simulink library "myLibrary"  (R2023a)
settings: Solver=VariableStepAuto  StartTime=0.0  StopTime=10.0  RelTol=1e-3
undefined symbols (not defined in the file): Cac_n1, ctrl1, Da, Discrete, dtha, ee_sli_rtmsupport, FA, gcbh, Ha, Ini, init_line, init_load, init_SG, init_TH, init_trafo, init_VSC, initMachineBlocks, Ka, Lf, Llkd_pu, Llkq1_pu, NET, P, plots_step, q0, Rac_n1, Radd, Rkd_pu, Rkq1_pu, Rload_add, sim_config, spsSteamTurbineModel, T_global, T_load, T_NET, T_SG, T_TH, T_trafo, T_VSC, Ts, tstep, V1
libraries: spsSeriesRLCBranchLib x57, spsParallelRLCBranchLib x39, eeGeneralControl x38, spsCurrentMeasurementLib x20, spsFirstOrderFilterLib x16, spsVoltageMeasurementLib x14, spsControlledVoltageSourceLib x12, $bdroot x9, dspsigops x6, spsThreePhaseVIMeasurementLib x5, spsPLL3phLib x4, spsThreePhaseBreakerLib x3
(part 1 of 7)
settings Model: Creator=CITCEA  LastModifiedBy=Francesca
settings DebuggingCC: UnconnectedInputMsg=warning  UnconnectedOutputMsg=warning  UnconnectedLineMsg=warning
settings ModelReferenceCC: EnableRefExpFcnMdlSchedulingChecks=on
settings RTWCC: DLArmComputeVersion=19.05

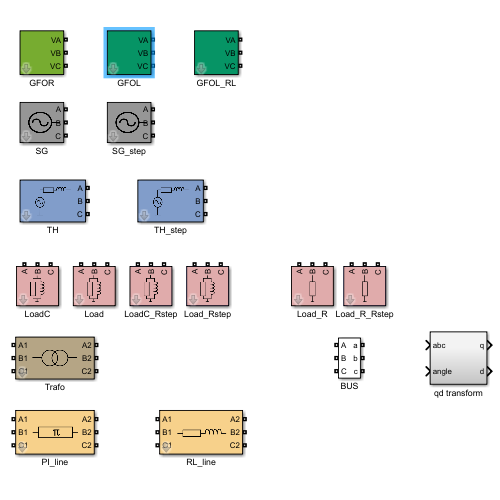
[thumbnail: Simulink's stored preview of the top-level diagram]
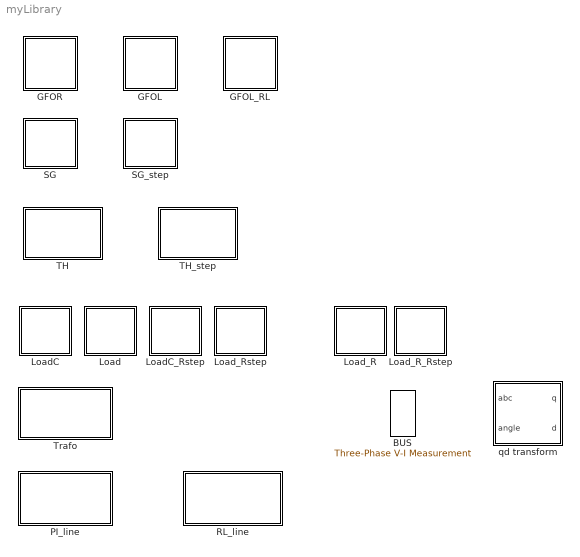
== system myLibrary ==
  BUS : spsThreePhaseVIMeasurementLib/Three-Phase V-I Measurement  VoltageMeasurement=phase-to-phase  SetLabelV=on  LabelV=V  Vpu=off  VpuLL=off  CurrentMeasurement=yes  SetLabelI=on  LabelI=I  Ipu=off  Pbase=100e6  Vbase=500e3  OutputType=Complex  PhasorSimulation=off  PSBequivalent=0
  GFOL : Subsystem  mask{T_VSC_global=T_VSC, initVSC_global=init_VSC, num=1}
      mask prompts: T_VSC_global "T_VSC"; initVSC_global "init_VSC"
      mask init:
      | T_VSC = T_VSC_global(num,:);
      | initVSC = initVSC_global{num};
      | 
      | set_param([gcb '/Control/Goto_w'],'GotoTag',['w_GFOL' num2str(num)])
      | set_param([gcb '/Control/From_w'],'GotoTag',['w_GFOL' num2str(num)])
  GFOL_RL : Subsystem  mask{T_VSC_global=T_VSC, initVSC_global=init_VSC, num=1}
      mask prompts: T_VSC_global "T_VSC"; initVSC_global "init_VSC"
      mask init:
      | T_VSC = T_VSC_global(num,:);
      | initVSC = initVSC_global{num};
      | 
      | set_param([gcb '/Control/Goto_w'],'GotoTag',['w_GFOL' num2str(num)])
      | set_param([gcb '/Control/From_w'],'GotoTag',['w_GFOL' num2str(num)])
  GFOR : Subsystem  mask{T_VSC_global=T_VSC, initVSC_global=init_VSC, num=1}
      mask prompts: T_VSC_global "T_VSC"; initVSC_global "init_VSC"
      mask init:
      | T_VSC = T_VSC_global(num,:);
      | initVSC = initVSC_global{num};
      | 
      | set_param([gcb '/Control/Goto_theta'],'GotoTag',['theta_GFOR' num2str(num)])
      | set_param([gcb '/Control/PLL/Goto_w'],'GotoTag',['w_GFOR' num2str(num)])
  Load : Subsystem  mask{T_load_global=T_load, initLoad_global=init_load, num=1}
      mask prompts: T_load_global "T_load"; initLoad_global "init_load"
      mask init:
      | T = T_load_global(num,:);
      | ini = initLoad_global{num};
      mask Display:
      | % Use specified image as mask icon
      | image('load.png')
  LoadC : Subsystem  mask{T_load_global=T_load, initLoad_global=init_load, num=1}
      mask prompts: T_load_global "T_load"; initLoad_global "init_load"
      mask init:
      | T = T_load_global(num,:);
      | ini = initLoad_global{num};
      mask Display:
      | % Use specified image as mask icon
      | image('load.png')
  LoadC_Rstep : Subsystem  mask{T_load_global=T_load, initLoad_global=init_load, num=1, tstep=tstep, Radd=Radd}
      mask prompts: T_load_global "T_load"; initLoad_global "init_load"
      mask init:
      | T = T_load_global(num,:);
      | ini = initLoad_global{num};
      mask Display:
      | % Use specified image as mask icon
      | image('load.png')
  Load_R : Subsystem  mask{T_load_global=T_load, num=1}
      mask prompts: T_load_global "T_load"
      mask init:
      | T = T_load_global(num,:);
      mask Display:
      | % Use specified image as mask icon
      | image('load_R.png')
  Load_R_Rstep : Subsystem  mask{T_load_global=T_load, num=1, tstep=tstep, Radd=Radd}
      mask prompts: T_load_global "T_load"
      mask init:
      | T = T_load_global(num,:);
      mask Display:
      | % Use specified image as mask icon
      | image('load_R.png')
  Load_Rstep : Subsystem  mask{T_load_global=T_load, initLoad_global=init_load, num=1, tstep=tstep, Radd=Radd}
      mask prompts: T_load_global "T_load"; initLoad_global "init_load"
      mask init:
      | T = T_load_global(num,:);
      | ini = initLoad_global{num};
      mask Display:
      | % Use specified image as mask icon
      | image('load.png')
  PI_line : Subsystem  mask{T_line_global=T_NET, initLine_global=init_line, num=1, set_C0=ones(1,6), set_iL0=0}
      mask prompts: T_line_global "T_line"; initLine_global "init_line"; set_C0 "init_cap"; set_iL0 "init_ind"
      mask init:
      | T = T_line_global(num,:);
      | ini = initLine_global{num};
      | set_C00 = set_C0(1,1);
      | set_C01 = set_C0(1,2);
      | set_C02 = set_C0(1,3);
      | set_C03 = set_C0(1,4);
      | set_C04 = set_C0(1,5);
      | set_C05 = set_C0(1,6);
      | set_param([gcb '/Series RLC Branch'],'Setx0',set_C00)
      | set_param([gcb '/Series RLC Branch1'],'Setx0',set_C01)
      | set_param([gcb '/Series RLC Branch2'],'Setx0',set_C02)
      | set_param([gcb '/Series RLC Branch3'],'Setx0',set_C03)
      | set_param([gcb '/Series RLC Branch4'],'Setx0',set_C04)
      | set_param([gcb '/Series RLC Branch5'],'Setx0',set_C05)
      | set_param([gcb '/Series RLC Branch6'],'SetiL0',set_iL0)
      mask Display:
      | % Use specified image as mask icon
      | image('PI.png')
  RL_line : Subsystem  mask{T_line_global=T_NET, initLine_global=init_line, num=1}
      mask prompts: T_line_global "T_line"; initLine_global "init_line"
      mask init:
      | T = T_line_global(num,:);
      | ini = initLine_global{num};
      mask Display:
      | % Use specified image as mask icon
      | image('RL.png')
  SG : Subsystem  mask{num=1, init_SG_global=init_SG, initMachineBlocks=initMachineBlocks, T_SG_global=T_SG}
      mask prompts: init_SG_global "init_SG"; initMachineBlocks "initMachine"; T_SG_global "T_SG"
      mask init:
      | initSG = init_SG_global{num};
      | T_SG = T_SG_global(num,:);
      | SGnum = num;
      | 
      | T_SG.exc = T_SG.exc{:};
      | T_SG.mech = T_SG.mech{:};
      | T_SG.PSS = T_SG.PSS{:};
      | 
      | 
      | switch T_SG.pss{:}
      |     case '2A'
      |         hasPSS = 1;
      |         set_param([gcb '/Exciter/PSS 2A'],'commented', 'off')
      |     case 'no'
      |         hasPSS = 0;
      |         set_param([gcb '/Exciter/PSS 2A'],'commented', 'on')
      | end
      | 
      | switch T_SG.govturb{:}
      |     case 'IEEEG1'
      |         selectGovturb= 1;
      |         set_param([gcb '/Governor-Turbine/IEEEG1'],'commented', 'off')
      |         set_param([gcb '/Governor-Turbine/Steam Turbine and Governor'],'commented', 'on')
      |     case 'TANDEM-SINGLE'
      |         selectGovturb= 2;
      |         T_SG.genType = 0;
      |         set_param([gcb '/Governor-Turbine/IEEEG1'],'commented', 'on')
      |         set_param([gcb '/Governor-Turbine/Steam Turbine and Governor'],'commented', 'off')
      |     case 'TANDEM-MULTI'
      |         selectGovturb= 2;
      |         T_SG.genType = 1;
      |         set_param([gcb '/Governor-Turbine/IEEEG1'],'commented', 'on')
      |         set_param([gcb '/Governor-Turbine/Steam Turbine and Governor'],'commented', 'off')
      |     case 'no'
      |         selectGovturb= 3;
      |         set_param([gcb '/Governor-Turbine/IEEEG1'],'commented', 'on')
      |         set_param([gcb '/Governor-Turbine/Steam Turbine and Governor'],'commented', 'on')
      | end
      | 
      | switch T_SG.exciter{:} 
      |     case 'AC4A'
      |         selectExciter = 1;
      |         set_param([gcb '/Exciter/Exciter AC4A'],'commented', 'off')
      |         set_param([gcb '/Exciter/Exciter ST4B'],'commented', 'on')
      |         set_param([gcb '/Exciter/Exciter ST1'],'commented', 'on')
      |     case 'ST4B'
      |         selectExciter = 2;
      |         set_param([gcb '/Exciter/Exciter AC4A'],'commented', 'on')
      |         set_param([gcb '/Exciter/Exciter ST4B'],'commented', 'off')
      |         set_param([gcb '/Exciter/Exciter ST1'],'commented', 'on')
      |     case 'ST1'
      |         selectExciter = 3;
      |         set_param([gcb '/Exciter/Exciter AC4A'],'commented', 'on')
      |         set_param([gcb '/Exciter/Exciter ST4B'],'commented', 'on')
      |         set_param([gcb '/Exciter/Exciter ST1'],'commented', 'off')
      |     case 'no'
      |         selectExciter = 4;
      |         set_param([gcb '/Exciter/Exciter AC4A'],'commented', 'on')
      |         set_param([gcb '/Exciter/Exciter ST4B'],'commented', 'on')
      |         set_param([gcb '/Exciter/Exciter ST1'],'commented', 'on')
      | end
      | 
      | set_param([gcb '/Goto_theta'],'GotoTag',['theta_SG' num2str(SGnum)])
      | set_param([gcb '/Goto_w'],'GotoTag',['w_SG' num2str(SGnum)])
      mask Display:
      | % Use specified image as mask icon
      | image('SG.png')
  SG_step : Subsystem  mask{num=1, init_SG_global=init_SG, initMachineBlocks=initMachineBlocks, T_SG_global=T_SG, step_var=Pref, tstep=sim_config.tstep}
      mask prompts: init_SG_global "init_SG"; initMachineBlocks "initMachine"; T_SG_global "T_SG"
      mask init:
      | initSG = init_SG_global{num};
      | T_SG = T_SG_global(num,:);
      | SGnum = num;
      | 
      | T_SG.exc = T_SG.exc{:};
      | T_SG.mech = T_SG.mech{:};
      | T_SG.PSS = T_SG.PSS{:};
      | 
      | 
      | switch T_SG.pss{:}
      |     case '2A'
      |         hasPSS = 1;
      |         set_param([gcb '/Exciter/PSS 2A'],'commented', 'off')
      |     case 'no'
      |         hasPSS = 0;
      |         set_param([gcb '/Exciter/PSS 2A'],'commented', 'on')
      | end
      | 
      | switch T_SG.govturb{:}
      |     case 'IEEEG1'
      |         selectGovturb= 1;
      |         set_param([gcb '/Governor-Turbine/IEEEG1'],'commented', 'off')
      |         set_param([gcb '/Governor-Turbine/Steam Turbine and Governor'],'commented', 'on')
      |     case 'TANDEM-SINGLE'
      |         selectGovturb= 2;
      |         T_SG.genType = 0;
      |         set_param([gcb '/Governor-Turbine/IEEEG1'],'commented', 'on')
      |         set_param([gcb '/Governor-Turbine/Steam Turbine and Governor'],'commented', 'off')
      |     case 'TANDEM-MULTI'
      |         selectGovturb= 2;
      |         T_SG.genType = 1;
      |         set_param([gcb '/Governor-Turbine/IEEEG1'],'commented', 'on')
      |         set_param([gcb '/Governor-Turbine/Steam Turbine and Governor'],'commented', 'off')
      |     case 'no'
      |         selectGovturb= 3;
      |         set_param([gcb '/Governor-Turbine/IEEEG1'],'commented', 'on')
      |         set_param([gcb '/Governor-Turbine/Steam Turbine and Governor'],'commented', 'on')
      | end
      | 
      | switch T_SG.exciter{:} 
      |     case 'AC4A'
      |         selectExciter = 1;
      |         set_param([gcb '/Exciter/Exciter AC4A'],'commented', 'off')
      |         set_param([gcb '/Exciter/Exciter ST4B'],'commented', 'on')
      |         set_param([gcb '/Exciter/Exciter ST1'],'commented', 'on')
      |     case 'ST4B'
      |         selectExciter = 2;
      |         set_param([gcb '/Exciter/Exciter AC4A'],'commented', 'on')
      |         set_param([gcb '/Exciter/Exciter ST4B'],'commented', 'off')
      |         set_param([gcb '/Exciter/Exciter ST1'],'commented', 'on')
      |     case 'ST1'
      |         selectExciter = 3;
      |         set_param([gcb '/Exciter/Exciter AC4A'],'commented', 'on')
      |         set_param([gcb '/Exciter/Exciter ST4B'],'commented', 'on')
      |         set_param([gcb '/Exciter/Exciter ST1'],'commented', 'off')
      |     case 'no'
      |         selectExciter = 4;
      |         set_param([gcb '/Exciter/Exciter AC4A'],'commented', 'on')
      |         set_param([gcb '/Exciter/Exciter ST4B'],'commented', 'on')
      |         set_param([gcb '/Exciter/Exciter ST1'],'commented', 'on')
      | end
      | 
      | set_param([gcb '/Goto_theta'],'GotoTag',['theta_SG' num2str(SGnum)])
      | set_param([gcb '/Goto_w'],'GotoTag',['w_SG' num2str(SGnum)])
      | 
      | switch step_var
      |     case 'Pref'
      |         tstep_P = tstep;
      |         tstep_V = 1e3;
      |     case 'Vref'
      |         tstep_P = 1e3;
      |         tstep_V = tstep;
      | end
      mask TypeOptions step_var: Pref | Vref
      mask Display:
      | % Use specified image as mask icon
      | image('SG.png')
  TH : Subsystem  mask{T_TH_global=T_TH, initTH_global=init_TH, num=1}
      mask prompts: T_TH_global "T_TH"; initTH_global "init_TH"
      mask init:
      | T = T_TH_global(num,:);
      | ini = initTH_global{num};
      mask Display:
      | port_label('rconn', 1, 'A')
      | port_label('rconn', 2, 'B')
      | port_label('rconn', 3, 'C')
      | 
      | % Use specified image as mask icon
      | image('TH.png')
  TH_step : Subsystem  mask{T_TH_global=T_TH, initTH_global=init_TH, num=1, tstep=tstep, V1=V1}
      mask prompts: T_TH_global "T_TH"; initTH_global "init_TH"
      mask init:
      | T = T_TH_global(num,:);
      | ini = initTH_global{num};
      mask Display:
      | port_label('rconn', 1, 'A')
      | port_label('rconn', 2, 'B')
      | port_label('rconn', 3, 'C')
      | 
      | % Use specified image as mask icon
      | image('TH.png')
  Trafo : Subsystem  mask{T_trafo_global=T_trafo, initTrafo_global=init_trafo, num=3}
      mask prompts: T_trafo_global "T_trafo"; initTrafo_global "init_trafo"
      mask init:
      | T = T_trafo_global(num,:);
      | ini = initTrafo_global{num};
      mask Display:
      | % Use specified image as mask icon
      | image('trafo.png')
  qd transform : Subsystem

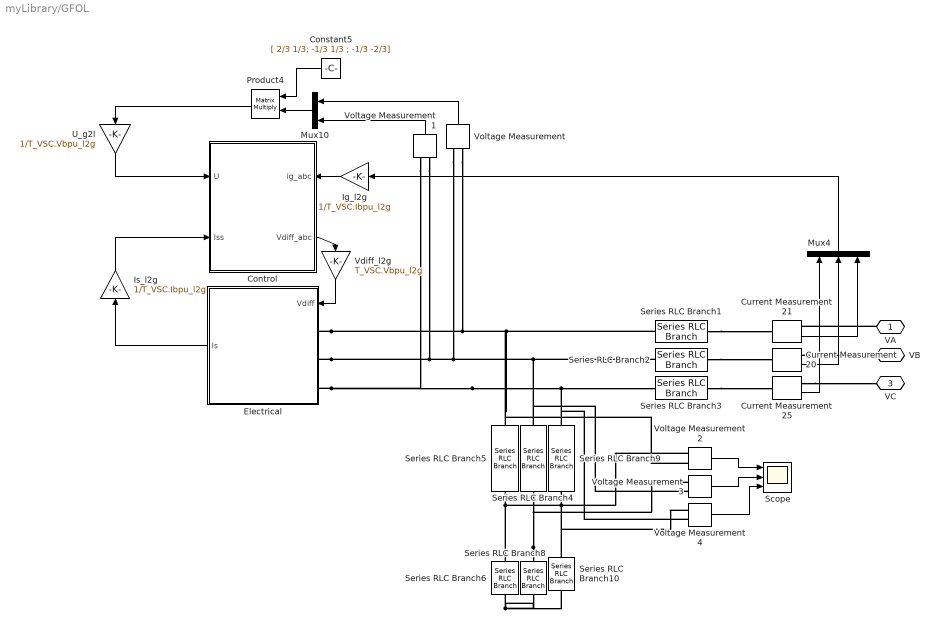
== system myLibrary/GFOL ==
  Constant5 : Constant  Value=[ 2/3 1/3; -1/3 1/3 ; -1/3 -2/3]
  Control : Subsystem
      settings: PortSchema="{\"entries\":[{\"content\":{\"sides\":[{\"content\":{},\"type\":\"ConnectorPlacement.EquallySpacedRectSide\",\"uuid\":\"681c0b5f-022d-4b6d-8fe2-73940743a76e\"},{\"content\":{\"side\":\"RIGHT\"},\"type\":\"ConnectorPlacement.EquallySpacedRectSide\",\"uuid\":\"e9b400c8-e13f-4caf-91a1-f348979675fd\"},{\"content\":{\"connectorIds\":[\"In1\",\"Out1\"],\"side\":\"TOP\"},\"type\":\"ConnectorPlacement.EquallySpacedRectSide\",\"uuid\":\"348007cb-ce67-4c45-ad7b-36ba89db6185\"},{\"content\":{\"connectorIds\":[\"In2\",\"In3\"],\"side\":\"BOTTOM\"},\"type\":\"ConnectorPlacement.EquallySpacedRectSide\",\"uuid\":\"fd6a847a-5d69-44cd-a0d1-495126761350\"}]},\"type\":\"ConnectorPlacement.EquallySpacedConnector\",\"uuid\":\"d16b8cae-5ced-4c76-a87e-983e154fb48f\"}],\"packageUris\":[\"http://schema.mathworks.com/mf0/Connector/R2020b\"],\"version\":\"1.0\"}"
  Current Measurement20 : spsCurrentMeasurementLib/Current Measurement  PhasorSimulation=off  OutputType=Complex  PSBequivalent=0
  Current Measurement21 : spsCurrentMeasurementLib/Current Measurement  PhasorSimulation=off  OutputType=Complex  PSBequivalent=0
  Current Measurement25 : spsCurrentMeasurementLib/Current Measurement  PhasorSimulation=off  OutputType=Complex  PSBequivalent=0
  Electrical : Subsystem
  Ig_l2g : Gain  Gain=1/T_VSC.Ibpu_l2g
  Is_l2g : Gain  Gain=1/T_VSC.Ibpu_l2g
  Mux10 : Mux  Inputs=2
  Mux4 : Mux  Inputs=3
  Product4 : Product  Multiplication=Matrix(*)
  Scope : Scope  NumInputPorts=3
  Series RLC Branch1 : spsSeriesRLCBranchLib/Series RLC Branch  LConnTagsString=__new0  RConnTagsString=__new0  BranchType=RL  Resistance=initVSC.Rtr  Inductance=initVSC.Ltr  SetiL0=off  InitialCurrent=initVSC.Iga  Capacitance=P.C  Setx0=on  InitialVoltage=P.C  Measurements=None
  Series RLC Branch10 : spsSeriesRLCBranchLib/Series RLC Branch  LConnTagsString=__new0  RConnTagsString=__new0  BranchType=R  Resistance=initVSC.Rac  Inductance=Lf  SetiL0=off  InitialCurrent=0  Capacitance=Cac_n1  Setx0=on  InitialVoltage=vcini_n1  Measurements=None
  Series RLC Branch2 : spsSeriesRLCBranchLib/Series RLC Branch  LConnTagsString=__new0  RConnTagsString=__new0  BranchType=RL  Resistance=initVSC.Rtr  Inductance=initVSC.Ltr  SetiL0=on  InitialCurrent=initVSC.Igb  Capacitance=P.C  Setx0=on  InitialVoltage=P.C  Measurements=None
  Series RLC Branch3 : spsSeriesRLCBranchLib/Series RLC Branch  LConnTagsString=__new0  RConnTagsString=__new0  BranchType=RL  Resistance=initVSC.Rtr  Inductance=initVSC.Ltr  SetiL0=on  InitialCurrent=initVSC.Igc  Capacitance=P.C  Setx0=on  InitialVoltage=P.C  Measurements=None
  Series RLC Branch4 : spsSeriesRLCBranchLib/Series RLC Branch  LConnTagsString=__new0  RConnTagsString=__new0  BranchType=C  Resistance=Rac_n1  Inductance=Lf  SetiL0=off  InitialCurrent=0  Capacitance=initVSC.Cac  Setx0=on  InitialVoltage=initVSC.Ucap_b  Measurements=None
  Series RLC Branch5 : spsSeriesRLCBranchLib/Series RLC Branch  LConnTagsString=__new0  RConnTagsString=__new0  BranchType=C  Resistance=Rac_n1  Inductance=Lf  SetiL0=off  InitialCurrent=0  Capacitance=initVSC.Cac  Setx0=on  InitialVoltage=initVSC.Ucap_a  Measurements=None
  Series RLC Branch6 : spsSeriesRLCBranchLib/Series RLC Branch  LConnTagsString=__new0  RConnTagsString=__new0  BranchType=R  Resistance=initVSC.Rac  Inductance=Lf  SetiL0=off  InitialCurrent=0  Capacitance=Cac_n1  Setx0=on  InitialVoltage=vcini_n1  Measurements=None
  Series RLC Branch8 : spsSeriesRLCBranchLib/Series RLC Branch  LConnTagsString=__new0  RConnTagsString=__new0  BranchType=R  Resistance=initVSC.Rac  Inductance=Lf  SetiL0=off  InitialCurrent=0  Capacitance=Cac_n1  Setx0=on  InitialVoltage=vcini_n1  Measurements=None
  Series RLC Branch9 : spsSeriesRLCBranchLib/Series RLC Branch  LConnTagsString=__new0  RConnTagsString=__new0  BranchType=C  Resistance=Rac_n1  Inductance=Lf  SetiL0=off  InitialCurrent=0  Capacitance=initVSC.Cac  Setx0=on  InitialVoltage=initVSC.Ucap_c  Measurements=None
  U_g2l : Gain  Gain=1/T_VSC.Vbpu_l2g
  Vdiff_l2g : Gain  Gain=T_VSC.Vbpu_l2g
  Voltage Measurement{,1..4} (5 alike) : spsVoltageMeasurementLib/Voltage Measurement  PhasorSimulation=off  OutputType=Complex  PSBequivalent=0
  VA : PMIOPort  Side=Right
  VB : PMIOPort  Port=2  Side=Right
  VC : PMIOPort  Port=3  Side=Right
  wires:
  Voltage Measurement4/1 -> Scope/3
  Voltage Measurement2/1 -> Scope/1
  Voltage Measurement3/1 -> Scope/2
  Ig_l2g/1 -> Control/1(ig_abc)
  Current Measurement25/1 -> Mux4/3
  Mux4/1 -> Ig_l2g/1
  Current Measurement21/1 -> Mux4/1
  Current Measurement20/1 -> Mux4/2
  U_g2l/1 -> Control/2(U)
  Is_l2g/1 -> Control/3(Iss)
  Vdiff_l2g/1 -> Electrical/1(Vdiff)
  Electrical/1(Is) -> Is_l2g/1
  Control/1(Vdiff_abc) -> Vdiff_l2g/1
  Product4/1 -> U_g2l/1
  Voltage Measurement/1 -> Mux10/1
  Mux10/1 -> Product4/2
  Constant5/1 -> Product4/1
  Voltage Measurement1/1 -> Mux10/2
  connections:
  Series RLC Branch6/RConn1 -- Series RLC Branch8/RConn1 -- Series RLC Branch10/RConn1
  Series RLC Branch9/RConn1 -- Series RLC Branch10/LConn1 -- Voltage Measurement4/LConn2
  Series RLC Branch8/LConn1 -- Series RLC Branch4/RConn1 -- Voltage Measurement3/LConn2
  Series RLC Branch5/RConn1 -- Series RLC Branch6/LConn1 -- Voltage Measurement2/LConn2
  Series RLC Branch3/RConn1 -- Current Measurement25/LConn1
  Series RLC Branch2/RConn1 -- Current Measurement20/LConn1
  Series RLC Branch1/RConn1 -- Current Measurement21/LConn1
  Current Measurement25/RConn1 -- VC/RConn1
  Electrical/LConn2 -- Voltage Measurement/LConn2 -- Series RLC Branch2/LConn1 -- Voltage Measurement3/LConn1 -- Series RLC Branch4/LConn1 -- Voltage Measurement1/LConn1
  VA/RConn1 -- Current Measurement21/RConn1
  Electrical/LConn3 -- Series RLC Branch3/LConn1 -- Voltage Measurement4/LConn1 -- Series RLC Branch9/LConn1 -- Voltage Measurement1/LConn2
  Electrical/LConn1 -- Voltage Measurement/LConn1 -- Voltage Measurement2/LConn1 -- Series RLC Branch5/LConn1 -- Series RLC Branch1/LConn1
  VB/RConn1 -- Current Measurement20/RConn1

== system myLibrary/GFOL_RL ==
  Constant5 : Constant  Value=[ 2/3 1/3; -1/3 1/3 ; -1/3 -2/3]
  Control : Subsystem
      settings: PortSchema="{\"entries\":[{\"content\":{\"sides\":[{\"content\":{\"connectorIds\":[]},\"type\":\"ConnectorPlacement.EquallySpacedRectSide\",\"uuid\":\"681c0b5f-022d-4b6d-8fe2-73940743a76e\"},{\"content\":{\"connectorIds\":[],\"side\":\"RIGHT\"},\"type\":\"ConnectorPlacement.EquallySpacedRectSide\",\"uuid\":\"e9b400c8-e13f-4caf-91a1-f348979675fd\"},{\"content\":{\"connectorIds\":[\"Out1\"],\"side\":\"TOP\"},\"type\":\"ConnectorPlacement.EquallySpacedRectSide\",\"uuid\":\"348007cb-ce67-4c45-ad7b-36ba89db6185\"},{\"content\":{\"connectorIds\":[\"In1\",\"In2\"],\"side\":\"BOTTOM\"},\"type\":\"ConnectorPlacement.EquallySpacedRectSide\",\"uuid\":\"fd6a847a-5d69-44cd-a0d1-495126761350\"}]},\"type\":\"ConnectorPlacement.EquallySpacedConnector\",\"uuid\":\"d16b8cae-5ced-4c76-a87e-983e154fb48f\"}],\"packageUris\":[\"http://schema.mathworks.com/mf0/Connector/R2020b\"],\"version\":\"1.0\"}"
  Electrical : Subsystem
  Is_l2g : Gain  Gain=1/T_VSC.Ibpu_l2g
  Mux10 : Mux  Inputs=2
  Product4 : Product  Multiplication=Matrix(*)
  Series RLC Branch1 : spsSeriesRLCBranchLib/Series RLC Branch  LConnTagsString=__new0  RConnTagsString=__new0  BranchType=RL  Resistance=initVSC.Rtr  Inductance=initVSC.Ltr  SetiL0=off  InitialCurrent=initVSC.Iga  Capacitance=P.C  Setx0=on  InitialVoltage=P.C  Measurements=None
  Series RLC Branch2 : spsSeriesRLCBranchLib/Series RLC Branch  LConnTagsString=__new0  RConnTagsString=__new0  BranchType=RL  Resistance=initVSC.Rtr  Inductance=initVSC.Ltr  SetiL0=on  InitialCurrent=initVSC.Igb  Capacitance=P.C  Setx0=on  InitialVoltage=P.C  Measurements=None
  Series RLC Branch3 : spsSeriesRLCBranchLib/Series RLC Branch  LConnTagsString=__new0  RConnTagsString=__new0  BranchType=RL  Resistance=initVSC.Rtr  Inductance=initVSC.Ltr  SetiL0=on  InitialCurrent=initVSC.Igc  Capacitance=P.C  Setx0=on  InitialVoltage=P.C  Measurements=None
  U_g2l : Gain  Gain=1/T_VSC.Vbpu_l2g
  Vdiff_l2g : Gain  Gain=T_VSC.Vbpu_l2g
  Voltage Measurement : spsVoltageMeasurementLib/Voltage Measurement  PhasorSimulation=off  OutputType=Complex  PSBequivalent=0
  Voltage Measurement1 : spsVoltageMeasurementLib/Voltage Measurement  PhasorSimulation=off  OutputType=Complex  PSBequivalent=0
  VA : PMIOPort  Side=Right
  VB : PMIOPort  Port=2  Side=Right
  VC : PMIOPort  Port=3  Side=Right
  wires:
  U_g2l/1 -> Control/1(U)
  Is_l2g/1 -> Control/2(Iss)
  Vdiff_l2g/1 -> Electrical/1(Vdiff)
  Electrical/1(Is) -> Is_l2g/1
  Control/1(Vdiff_abc) -> Vdiff_l2g/1
  Product4/1 -> U_g2l/1
  Voltage Measurement/1 -> Mux10/1
  Mux10/1 -> Product4/2
  Constant5/1 -> Product4/1
  Voltage Measurement1/1 -> Mux10/2
  connections:
  Series RLC Branch3/RConn1 -- VC/RConn1
  Voltage Measurement/LConn2 -- Series RLC Branch2/LConn1 -- Voltage Measurement1/LConn1 -- Electrical/LConn2
  VA/RConn1 -- Series RLC Branch1/RConn1
  Electrical/LConn3 -- Series RLC Branch3/LConn1 -- Voltage Measurement1/LConn2
  Series RLC Branch1/LConn1 -- Voltage Measurement/LConn1 -- Electrical/LConn1
  VB/RConn1 -- Series RLC Branch2/RConn1

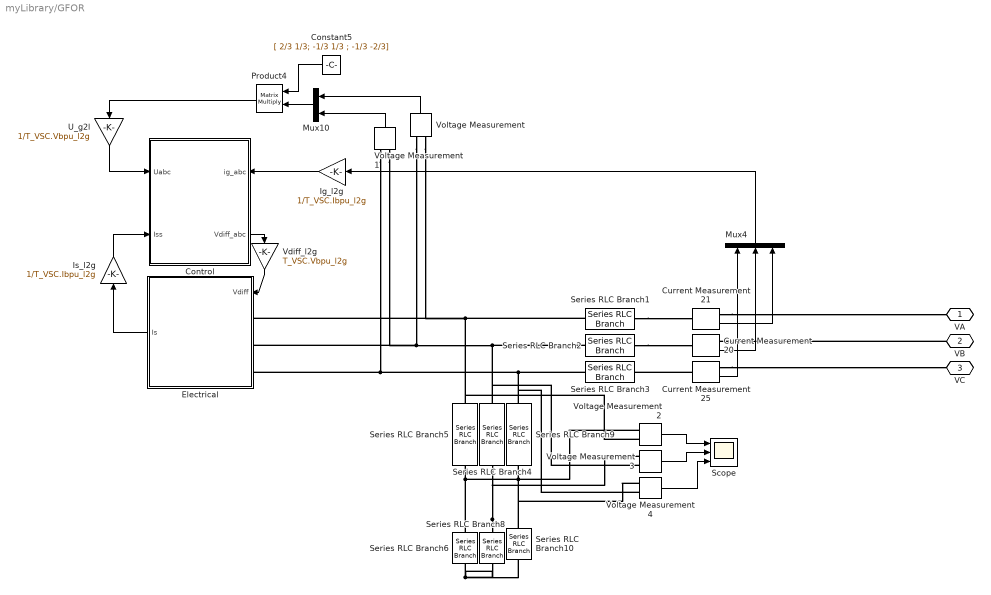
== system myLibrary/GFOR ==
  Constant5 : Constant  Value=[ 2/3 1/3; -1/3 1/3 ; -1/3 -2/3]
  Control : Subsystem
      settings: PortSchema="{\"entries\":[{\"content\":{\"sides\":[{\"content\":{},\"type\":\"ConnectorPlacement.EquallySpacedRectSide\",\"uuid\":\"681c0b5f-022d-4b6d-8fe2-73940743a76e\"},{\"content\":{\"side\":\"RIGHT\"},\"type\":\"ConnectorPlacement.EquallySpacedRectSide\",\"uuid\":\"e9b400c8-e13f-4caf-91a1-f348979675fd\"},{\"content\":{\"connectorIds\":[\"In1\",\"Out1\"],\"side\":\"TOP\"},\"type\":\"ConnectorPlacement.EquallySpacedRectSide\",\"uuid\":\"348007cb-ce67-4c45-ad7b-36ba89db6185\"},{\"content\":{\"connectorIds\":[\"In2\",\"In3\"],\"side\":\"BOTTOM\"},\"type\":\"ConnectorPlacement.EquallySpacedRectSide\",\"uuid\":\"fd6a847a-5d69-44cd-a0d1-495126761350\"}]},\"type\":\"ConnectorPlacement.EquallySpacedConnector\",\"uuid\":\"d16b8cae-5ced-4c76-a87e-983e154fb48f\"}],\"packageUris\":[\"http://schema.mathworks.com/mf0/Connector/R2020b\"],\"version\":\"1.0\"}"
  Current Measurement20 : spsCurrentMeasurementLib/Current Measurement  PhasorSimulation=off  OutputType=Complex  PSBequivalent=0
  Current Measurement21 : spsCurrentMeasurementLib/Current Measurement  PhasorSimulation=off  OutputType=Complex  PSBequivalent=0
  Current Measurement25 : spsCurrentMeasurementLib/Current Measurement  PhasorSimulation=off  OutputType=Complex  PSBequivalent=0
  Electrical : Subsystem
  Ig_l2g : Gain  Gain=1/T_VSC.Ibpu_l2g
  Is_l2g : Gain  Gain=1/T_VSC.Ibpu_l2g
  Mux10 : Mux  Inputs=2
  Mux4 : Mux  Inputs=3
  Product4 : Product  Multiplication=Matrix(*)
  Scope : Scope  NumInputPorts=3
  Series RLC Branch1 : spsSeriesRLCBranchLib/Series RLC Branch  LConnTagsString=__new0  RConnTagsString=__new0  BranchType=RL  Resistance=initVSC.Rtr  Inductance=initVSC.Ltr  SetiL0=off  InitialCurrent=initVSC.Iga  Capacitance=P.C  Setx0=on  InitialVoltage=P.C  Measurements=None
  Series RLC Branch10 : spsSeriesRLCBranchLib/Series RLC Branch  LConnTagsString=__new0  RConnTagsString=__new0  BranchType=R  Resistance=initVSC.Rac  Inductance=Lf  SetiL0=off  InitialCurrent=0  Capacitance=Cac_n1  Setx0=on  InitialVoltage=vcini_n1  Measurements=None
  Series RLC Branch2 : spsSeriesRLCBranchLib/Series RLC Branch  LConnTagsString=__new0  RConnTagsString=__new0  BranchType=RL  Resistance=initVSC.Rtr  Inductance=initVSC.Ltr  SetiL0=on  InitialCurrent=initVSC.Igb  Capacitance=P.C  Setx0=on  InitialVoltage=P.C  Measurements=None
  Series RLC Branch3 : spsSeriesRLCBranchLib/Series RLC Branch  LConnTagsString=__new0  RConnTagsString=__new0  BranchType=RL  Resistance=initVSC.Rtr  Inductance=initVSC.Ltr  SetiL0=on  InitialCurrent=initVSC.Igc  Capacitance=P.C  Setx0=on  InitialVoltage=P.C  Measurements=None
  Series RLC Branch4 : spsSeriesRLCBranchLib/Series RLC Branch  LConnTagsString=__new0  RConnTagsString=__new0  BranchType=C  Resistance=Rac_n1  Inductance=Lf  SetiL0=off  InitialCurrent=0  Capacitance=initVSC.Cac  Setx0=on  InitialVoltage=initVSC.Ucap_b  Measurements=None
  Series RLC Branch5 : spsSeriesRLCBranchLib/Series RLC Branch  LConnTagsString=__new0  RConnTagsString=__new0  BranchType=C  Resistance=Rac_n1  Inductance=Lf  SetiL0=off  InitialCurrent=0  Capacitance=initVSC.Cac  Setx0=on  InitialVoltage=initVSC.Ucap_a  Measurements=None
  Series RLC Branch6 : spsSeriesRLCBranchLib/Series RLC Branch  LConnTagsString=__new0  RConnTagsString=__new0  BranchType=R  Resistance=initVSC.Rac  Inductance=Lf  SetiL0=off  InitialCurrent=0  Capacitance=Cac_n1  Setx0=on  InitialVoltage=vcini_n1  Measurements=None
  Series RLC Branch8 : spsSeriesRLCBranchLib/Series RLC Branch  LConnTagsString=__new0  RConnTagsString=__new0  BranchType=R  Resistance=initVSC.Rac  Inductance=Lf  SetiL0=off  InitialCurrent=0  Capacitance=Cac_n1  Setx0=on  InitialVoltage=vcini_n1  Measurements=None
  Series RLC Branch9 : spsSeriesRLCBranchLib/Series RLC Branch  LConnTagsString=__new0  RConnTagsString=__new0  BranchType=C  Resistance=Rac_n1  Inductance=Lf  SetiL0=off  InitialCurrent=0  Capacitance=initVSC.Cac  Setx0=on  InitialVoltage=initVSC.Ucap_c  Measurements=None
  U_g2l : Gain  Gain=1/T_VSC.Vbpu_l2g
  Vdiff_l2g : Gain  Gain=T_VSC.Vbpu_l2g
  Voltage Measurement{,1..4} (5 alike) : spsVoltageMeasurementLib/Voltage Measurement  PhasorSimulation=off  OutputType=Complex  PSBequivalent=0
  VA : PMIOPort  Side=Right
  VB : PMIOPort  Port=2  Side=Right
  VC : PMIOPort  Port=3  Side=Right
  wires:
  U_g2l/1 -> Control/2(Uabc)
  Vdiff_l2g/1 -> Electrical/1(Vdiff)
  Ig_l2g/1 -> Control/1(ig_abc)
  Is_l2g/1 -> Control/3(Iss)
  Voltage Measurement4/1 -> Scope/3
  Voltage Measurement3/1 -> Scope/2
  Voltage Measurement2/1 -> Scope/1
  Voltage Measurement1/1 -> Mux10/2
  Constant5/1 -> Product4/1
  Mux10/1 -> Product4/2
  Voltage Measurement/1 -> Mux10/1
  Product4/1 -> U_g2l/1
  Control/1(Vdiff_abc) -> Vdiff_l2g/1
  Electrical/1(Is) -> Is_l2g/1
  Current Measurement21/1 -> Mux4/1
  Mux4/1 -> Ig_l2g/1
  Current Measurement25/1 -> Mux4/3
  Current Measurement20/1 -> Mux4/2
  connections:
  Series RLC Branch1/LConn1 -- Series RLC Branch5/LConn1 -- Voltage Measurement2/LConn1 -- Voltage Measurement/LConn1 -- Electrical/LConn1
  Series RLC Branch2/LConn1 -- Series RLC Branch4/LConn1 -- Voltage Measurement3/LConn1 -- Voltage Measurement1/LConn1 -- Electrical/LConn2 -- Voltage Measurement/LConn2
  Series RLC Branch3/LConn1 -- Series RLC Branch9/LConn1 -- Voltage Measurement4/LConn1 -- Voltage Measurement1/LConn2 -- Electrical/LConn3
  Current Measurement21/RConn1 -- VA/RConn1
  Current Measurement25/RConn1 -- VC/RConn1
  VB/RConn1 -- Current Measurement20/RConn1
  Current Measurement25/LConn1 -- Series RLC Branch3/RConn1
  Series RLC Branch2/RConn1 -- Current Measurement20/LConn1
  Series RLC Branch1/RConn1 -- Current Measurement21/LConn1
  Series RLC Branch6/RConn1 -- Series RLC Branch10/RConn1 -- Series RLC Branch8/RConn1
  Series RLC Branch5/RConn1 -- Voltage Measurement2/LConn2 -- Series RLC Branch6/LConn1
  Series RLC Branch9/RConn1 -- Voltage Measurement4/LConn2 -- Series RLC Branch10/LConn1
  Series RLC Branch8/LConn1 -- Voltage Measurement3/LConn2 -- Series RLC Branch4/RConn1

== system myLibrary/Load ==
  Parallel RLC Branch : spsParallelRLCBranchLib/Parallel RLC Branch  LConnTagsString=a  RConnTagsString=__new0  BranchType=R  Resistance=T.R  Inductance=P.L  SetiL0=on  InitialCurrent=Ini.Ia*10  Capacitance=1e-6  Setx0=off  InitialVoltage=0  Measurements=None
  Parallel RLC Branch1 : spsParallelRLCBranchLib/Parallel RLC Branch  LConnTagsString=a  RConnTagsString=__new0  BranchType=R  Resistance=T.R  Inductance=P.L  SetiL0=on  InitialCurrent=Ini.Ia*10  Capacitance=1e-6  Setx0=off  InitialVoltage=0  Measurements=None
  Parallel RLC Branch2 : spsParallelRLCBranchLib/Parallel RLC Branch  LConnTagsString=a  RConnTagsString=__new0  BranchType=L  Resistance=P.R  Inductance=T.L  SetiL0=on  InitialCurrent=ini.Ib  Capacitance=1e-6  Setx0=off  InitialVoltage=0  Measurements=None
  Parallel RLC Branch3 : spsParallelRLCBranchLib/Parallel RLC Branch  LConnTagsString=a  RConnTagsString=__new0  BranchType=L  Resistance=P.R  Inductance=T.L  SetiL0=on  InitialCurrent=ini.Ia  Capacitance=1e-6  Setx0=off  InitialVoltage=0  Measurements=None
  Parallel RLC Branch4 : spsParallelRLCBranchLib/Parallel RLC Branch  LConnTagsString=a  RConnTagsString=__new0  BranchType=R  Resistance=T.R  Inductance=P.L  SetiL0=on  InitialCurrent=Ini.Ia*10  Capacitance=1e-6  Setx0=off  InitialVoltage=0  Measurements=None
  Parallel RLC Branch5 : spsParallelRLCBranchLib/Parallel RLC Branch  LConnTagsString=a  RConnTagsString=__new0  BranchType=L  Resistance=P.R  Inductance=T.L  SetiL0=on  InitialCurrent=ini.Ic  Capacitance=1e-6  Setx0=off  InitialVoltage=0  Measurements=None
  A : PMIOPort  Side=Left
  B : PMIOPort  Port=2  Side=Left
  C : PMIOPort  Port=3  Side=Left
  connections:
  Parallel RLC Branch2/LConn1 -- Parallel RLC Branch1/RConn1 -- Parallel RLC Branch3/LConn1 -- Parallel RLC Branch/RConn1 -- Parallel RLC Branch4/RConn1 -- Parallel RLC Branch5/LConn1
  A/RConn1 -- Parallel RLC Branch3/RConn1 -- Parallel RLC Branch/LConn1
  Parallel RLC Branch1/LConn1 -- B/RConn1 -- Parallel RLC Branch2/RConn1
  C/RConn1 -- Parallel RLC Branch5/RConn1 -- Parallel RLC Branch4/LConn1

== system myLibrary/LoadC ==
  Parallel RLC Branch : spsParallelRLCBranchLib/Parallel RLC Branch  LConnTagsString=a  RConnTagsString=__new0  BranchType=R  Resistance=T.R  Inductance=P.L  SetiL0=on  InitialCurrent=Ini.Ia*10  Capacitance=1e-6  Setx0=off  InitialVoltage=0  Measurements=None
  Parallel RLC Branch1 : spsParallelRLCBranchLib/Parallel RLC Branch  LConnTagsString=a  RConnTagsString=__new0  BranchType=R  Resistance=T.R  Inductance=P.L  SetiL0=on  InitialCurrent=Ini.Ia*10  Capacitance=1e-6  Setx0=off  InitialVoltage=0  Measurements=None
  Parallel RLC Branch2 : spsParallelRLCBranchLib/Parallel RLC Branch  LConnTagsString=a  RConnTagsString=__new0  BranchType=C  Resistance=T.R  Inductance=P.L  SetiL0=on  InitialCurrent=Ini.Ia*10  Capacitance=T.C  Setx0=on  InitialVoltage=ini.Va  Measurements=None
  Parallel RLC Branch3 : spsParallelRLCBranchLib/Parallel RLC Branch  LConnTagsString=a  RConnTagsString=__new0  BranchType=C  Resistance=T.R  Inductance=P.L  SetiL0=on  InitialCurrent=Ini.Ia*10  Capacitance=T.C  Setx0=on  InitialVoltage=ini.Vb  Measurements=None
  Parallel RLC Branch4 : spsParallelRLCBranchLib/Parallel RLC Branch  LConnTagsString=a  RConnTagsString=__new0  BranchType=R  Resistance=T.R  Inductance=P.L  SetiL0=on  InitialCurrent=Ini.Ia*10  Capacitance=1e-6  Setx0=off  InitialVoltage=0  Measurements=None
  Parallel RLC Branch5 : spsParallelRLCBranchLib/Parallel RLC Branch  LConnTagsString=a  RConnTagsString=__new0  BranchType=C  Resistance=T.R  Inductance=P.L  SetiL0=on  InitialCurrent=Ini.Ia*10  Capacitance=T.C  Setx0=on  InitialVoltage=ini.Vc  Measurements=None
  A : PMIOPort  Side=Left
  B : PMIOPort  Port=2  Side=Left
  C : PMIOPort  Port=3  Side=Left
  connections:
  Parallel RLC Branch1/RConn1 -- Parallel RLC Branch3/RConn1 -- Parallel RLC Branch2/RConn1 -- Parallel RLC Branch/RConn1 -- Parallel RLC Branch5/RConn1 -- Parallel RLC Branch4/RConn1
  A/RConn1 -- Parallel RLC Branch2/LConn1 -- Parallel RLC Branch/LConn1
  Parallel RLC Branch1/LConn1 -- Parallel RLC Branch3/LConn1 -- B/RConn1
  C/RConn1 -- Parallel RLC Branch5/LConn1 -- Parallel RLC Branch4/LConn1

== system myLibrary/LoadC_Rstep ==
  Parallel RLC Branch : spsParallelRLCBranchLib/Parallel RLC Branch  LConnTagsString=a  RConnTagsString=__new0  BranchType=R  Resistance=T.R  Inductance=P.L  SetiL0=on  InitialCurrent=Ini.Ia*10  Capacitance=1e-6  Setx0=off  InitialVoltage=0  Measurements=None
  Parallel RLC Branch1 : spsParallelRLCBranchLib/Parallel RLC Branch  LConnTagsString=a  RConnTagsString=__new0  BranchType=R  Resistance=T.R  Inductance=P.L  SetiL0=on  InitialCurrent=Ini.Ia*10  Capacitance=1e-6  Setx0=off  InitialVoltage=0  Measurements=None
  Parallel RLC Branch10 : spsParallelRLCBranchLib/Parallel RLC Branch  LConnTagsString=a  RConnTagsString=__new0  BranchType=R  Resistance=Rload_add  Inductance=P.L  SetiL0=on  InitialCurrent=Ini.Ia*10  Capacitance=1e-6  Setx0=off  InitialVoltage=0  Measurements=None
  Parallel RLC Branch2 : spsParallelRLCBranchLib/Parallel RLC Branch  LConnTagsString=a  RConnTagsString=__new0  BranchType=C  Resistance=T.R  Inductance=P.L  SetiL0=on  InitialCurrent=Ini.Ia*10  Capacitance=T.C  Setx0=on  InitialVoltage=ini.Va  Measurements=None
  Parallel RLC Branch3 : spsParallelRLCBranchLib/Parallel RLC Branch  LConnTagsString=a  RConnTagsString=__new0  BranchType=C  Resistance=T.R  Inductance=P.L  SetiL0=on  InitialCurrent=Ini.Ia*10  Capacitance=T.C  Setx0=on  InitialVoltage=ini.Vb  Measurements=None
  Parallel RLC Branch4 : spsParallelRLCBranchLib/Parallel RLC Branch  LConnTagsString=a  RConnTagsString=__new0  BranchType=R  Resistance=T.R  Inductance=P.L  SetiL0=on  InitialCurrent=Ini.Ia*10  Capacitance=1e-6  Setx0=off  InitialVoltage=0  Measurements=None
  Parallel RLC Branch5 : spsParallelRLCBranchLib/Parallel RLC Branch  LConnTagsString=a  RConnTagsString=__new0  BranchType=C  Resistance=T.R  Inductance=P.L  SetiL0=on  InitialCurrent=Ini.Ia*10  Capacitance=T.C  Setx0=on  InitialVoltage=ini.Vc  Measurements=None
  Parallel RLC Branch6 : spsParallelRLCBranchLib/Parallel RLC Branch  LConnTagsString=a  RConnTagsString=__new0  BranchType=R  Resistance=Rload_add  Inductance=P.L  SetiL0=on  InitialCurrent=Ini.Ia*10  Capacitance=1e-6  Setx0=off  InitialVoltage=0  Measurements=None
  Parallel RLC Branch7 : spsParallelRLCBranchLib/Parallel RLC Branch  LConnTagsString=a  RConnTagsString=__new0  BranchType=R  Resistance=Rload_add  Inductance=P.L  SetiL0=on  InitialCurrent=Ini.Ia*10  Capacitance=1e-6  Setx0=off  InitialVoltage=0  Measurements=None
  Three-Phase Breaker : spsThreePhaseBreakerLib/Three-Phase Breaker  InitialState=open  SwitchA=on  SwitchB=on  SwitchC=on  SwitchTimes=[tstep 1e6]  External=off  BreakerResistance=1e-10  SnubberResistance=inf  SnubberCapacitance=inf  Measurements=None
  A : PMIOPort  Side=Left
  B : PMIOPort  Port=2  Side=Left
  C : PMIOPort  Port=3  Side=Left
  connections:
  Three-Phase Breaker/RConn3 -- Parallel RLC Branch10/LConn1
  Three-Phase Breaker/RConn2 -- Parallel RLC Branch7/LConn1
  Three-Phase Breaker/RConn1 -- Parallel RLC Branch6/LConn1
  Parallel RLC Branch10/RConn1 -- Parallel RLC Branch7/RConn1 -- Parallel RLC Branch6/RConn1 -- Parallel RLC Branch4/RConn1 -- Parallel RLC Branch2/RConn1 -- Parallel RLC Branch/RConn1 -- Parallel RLC Branch3/RConn1 -- Parallel RLC Branch1/RConn1 -- Parallel RLC Branch5/RConn1
  Parallel RLC Branch4/LConn1 -- Parallel RLC Branch5/LConn1 -- C/RConn1 -- Three-Phase Breaker/LConn3
  Parallel RLC Branch1/LConn1 -- Parallel RLC Branch3/LConn1 -- B/RConn1 -- Three-Phase Breaker/LConn2
  Parallel RLC Branch/LConn1 -- Parallel RLC Branch2/LConn1 -- A/RConn1 -- Three-Phase Breaker/LConn1

== system myLibrary/Load_R ==
  Parallel RLC Branch : spsParallelRLCBranchLib/Parallel RLC Branch  LConnTagsString=a  RConnTagsString=__new0  BranchType=R  Resistance=T.R  Inductance=P.L  SetiL0=on  InitialCurrent=Ini.Ia*10  Capacitance=1e-6  Setx0=off  InitialVoltage=0  Measurements=None
  Parallel RLC Branch1 : spsParallelRLCBranchLib/Parallel RLC Branch  LConnTagsString=a  RConnTagsString=__new0  BranchType=R  Resistance=T.R  Inductance=P.L  SetiL0=on  InitialCurrent=Ini.Ia*10  Capacitance=1e-6  Setx0=off  InitialVoltage=0  Measurements=None
  Parallel RLC Branch4 : spsParallelRLCBranchLib/Parallel RLC Branch  LConnTagsString=a  RConnTagsString=__new0  BranchType=R  Resistance=T.R  Inductance=P.L  SetiL0=on  InitialCurrent=Ini.Ia*10  Capacitance=1e-6  Setx0=off  InitialVoltage=0  Measurements=None
  A : PMIOPort  Side=Left
  B : PMIOPort  Port=2  Side=Left
  C : PMIOPort  Port=3  Side=Left
  connections:
  Parallel RLC Branch1/RConn1 -- Parallel RLC Branch4/RConn1 -- Parallel RLC Branch/RConn1
  Parallel RLC Branch/LConn1 -- A/RConn1
  Parallel RLC Branch1/LConn1 -- B/RConn1
  Parallel RLC Branch4/LConn1 -- C/RConn1

== system myLibrary/Load_R_Rstep ==
  Parallel RLC Branch : spsParallelRLCBranchLib/Parallel RLC Branch  LConnTagsString=a  RConnTagsString=__new0  BranchType=R  Resistance=T.R  Inductance=P.L  SetiL0=on  InitialCurrent=Ini.Ia*10  Capacitance=1e-6  Setx0=off  InitialVoltage=0  Measurements=None
  Parallel RLC Branch1 : spsParallelRLCBranchLib/Parallel RLC Branch  LConnTagsString=a  RConnTagsString=__new0  BranchType=R  Resistance=T.R  Inductance=P.L  SetiL0=on  InitialCurrent=Ini.Ia*10  Capacitance=1e-6  Setx0=off  InitialVoltage=0  Measurements=None
  Parallel RLC Branch10 : spsParallelRLCBranchLib/Parallel RLC Branch  LConnTagsString=a  RConnTagsString=__new0  BranchType=R  Resistance=Rload_add  Inductance=P.L  SetiL0=on  InitialCurrent=Ini.Ia*10  Capacitance=1e-6  Setx0=off  InitialVoltage=0  Measurements=None
  Parallel RLC Branch4 : spsParallelRLCBranchLib/Parallel RLC Branch  LConnTagsString=a  RConnTagsString=__new0  BranchType=R  Resistance=T.R  Inductance=P.L  SetiL0=on  InitialCurrent=Ini.Ia*10  Capacitance=1e-6  Setx0=off  InitialVoltage=0  Measurements=None
  Parallel RLC Branch6 : spsParallelRLCBranchLib/Parallel RLC Branch  LConnTagsString=a  RConnTagsString=__new0  BranchType=R  Resistance=Rload_add  Inductance=P.L  SetiL0=on  InitialCurrent=Ini.Ia*10  Capacitance=1e-6  Setx0=off  InitialVoltage=0  Measurements=None
  Parallel RLC Branch7 : spsParallelRLCBranchLib/Parallel RLC Branch  LConnTagsString=a  RConnTagsString=__new0  BranchType=R  Resistance=Rload_add  Inductance=P.L  SetiL0=on  InitialCurrent=Ini.Ia*10  Capacitance=1e-6  Setx0=off  InitialVoltage=0  Measurements=None
  Three-Phase Breaker : spsThreePhaseBreakerLib/Three-Phase Breaker  InitialState=open  SwitchA=on  SwitchB=on  SwitchC=on  SwitchTimes=[tstep 1e6]  External=off  BreakerResistance=1e-10  SnubberResistance=inf  SnubberCapacitance=inf  Measurements=None
  A : PMIOPort  Side=Left
  B : PMIOPort  Port=2  Side=Left
  C : PMIOPort  Port=3  Side=Left
  connections:
  Three-Phase Breaker/LConn1 -- Parallel RLC Branch/LConn1 -- A/RConn1
  Parallel RLC Branch1/LConn1 -- Three-Phase Breaker/LConn2 -- B/RConn1
  Three-Phase Breaker/LConn3 -- Parallel RLC Branch4/LConn1 -- C/RConn1
  Parallel RLC Branch1/RConn1 -- Parallel RLC Branch/RConn1 -- Parallel RLC Branch6/RConn1 -- Parallel RLC Branch7/RConn1 -- Parallel RLC Branch10/RConn1 -- Parallel RLC Branch4/RConn1
  Three-Phase Breaker/RConn1 -- Parallel RLC Branch6/LConn1
  Three-Phase Breaker/RConn2 -- Parallel RLC Branch7/LConn1
  Three-Phase Breaker/RConn3 -- Parallel RLC Branch10/LConn1

== system myLibrary/Load_Rstep ==
  Parallel RLC Branch : spsParallelRLCBranchLib/Parallel RLC Branch  LConnTagsString=a  RConnTagsString=__new0  BranchType=R  Resistance=T.R  Inductance=P.L  SetiL0=on  InitialCurrent=Ini.Ia*10  Capacitance=1e-6  Setx0=off  InitialVoltage=0  Measurements=None
  Parallel RLC Branch1 : spsParallelRLCBranchLib/Parallel RLC Branch  LConnTagsString=a  RConnTagsString=__new0  BranchType=R  Resistance=T.R  Inductance=P.L  SetiL0=on  InitialCurrent=Ini.Ia*10  Capacitance=1e-6  Setx0=off  InitialVoltage=0  Measurements=None
  Parallel RLC Branch10 : spsParallelRLCBranchLib/Parallel RLC Branch  LConnTagsString=a  RConnTagsString=__new0  BranchType=R  Resistance=Rload_add  Inductance=P.L  SetiL0=on  InitialCurrent=Ini.Ia*10  Capacitance=1e-6  Setx0=off  InitialVoltage=0  Measurements=None
  Parallel RLC Branch2 : spsParallelRLCBranchLib/Parallel RLC Branch  LConnTagsString=a  RConnTagsString=__new0  BranchType=L  Resistance=P.R  Inductance=T.L  SetiL0=on  InitialCurrent=ini.Ib  Capacitance=1e-6  Setx0=off  InitialVoltage=0  Measurements=None
  Parallel RLC Branch3 : spsParallelRLCBranchLib/Parallel RLC Branch  LConnTagsString=a  RConnTagsString=__new0  BranchType=L  Resistance=P.R  Inductance=T.L  SetiL0=on  InitialCurrent=ini.Ia  Capacitance=1e-6  Setx0=off  InitialVoltage=0  Measurements=None
  Parallel RLC Branch4 : spsParallelRLCBranchLib/Parallel RLC Branch  LConnTagsString=a  RConnTagsString=__new0  BranchType=R  Resistance=T.R  Inductance=P.L  SetiL0=on  InitialCurrent=Ini.Ia*10  Capacitance=1e-6  Setx0=off  InitialVoltage=0  Measurements=None
  Parallel RLC Branch5 : spsParallelRLCBranchLib/Parallel RLC Branch  LConnTagsString=a  RConnTagsString=__new0  BranchType=L  Resistance=P.R  Inductance=T.L  SetiL0=on  InitialCurrent=ini.Ic  Capacitance=1e-6  Setx0=off  InitialVoltage=0  Measurements=None
  Parallel RLC Branch6 : spsParallelRLCBranchLib/Parallel RLC Branch  LConnTagsString=a  RConnTagsString=__new0  BranchType=R  Resistance=Rload_add  Inductance=P.L  SetiL0=on  InitialCurrent=Ini.Ia*10  Capacitance=1e-6  Setx0=off  InitialVoltage=0  Measurements=None
  Parallel RLC Branch7 : spsParallelRLCBranchLib/Parallel RLC Branch  LConnTagsString=a  RConnTagsString=__new0  BranchType=R  Resistance=Rload_add  Inductance=P.L  SetiL0=on  InitialCurrent=Ini.Ia*10  Capacitance=1e-6  Setx0=off  InitialVoltage=0  Measurements=None
  Three-Phase Breaker : spsThreePhaseBreakerLib/Three-Phase Breaker  InitialState=open  SwitchA=on  SwitchB=on  SwitchC=on  SwitchTimes=[tstep 1e6]  External=off  BreakerResistance=1e-10  SnubberResistance=inf  SnubberCapacitance=inf  Measurements=None
  A : PMIOPort  Side=Left
  B : PMIOPort  Port=2  Side=Left
  C : PMIOPort  Port=3  Side=Left
  connections:
  Three-Phase Breaker/LConn1 -- A/RConn1 -- Parallel RLC Branch3/RConn1 -- Parallel RLC Branch/LConn1
  Parallel RLC Branch1/LConn1 -- Three-Phase Breaker/LConn2 -- B/RConn1 -- Parallel RLC Branch2/RConn1
  Three-Phase Breaker/LConn3 -- C/RConn1 -- Parallel RLC Branch5/RConn1 -- Parallel RLC Branch4/LConn1
  Parallel RLC Branch2/LConn1 -- Parallel RLC Branch1/RConn1 -- Parallel RLC Branch3/LConn1 -- Parallel RLC Branch/RConn1 -- Parallel RLC Branch4/RConn1 -- Parallel RLC Branch5/LConn1 -- Parallel RLC Branch6/RConn1 -- Parallel RLC Branch7/RConn1 -- Parallel RLC Branch10/RConn1
  Three-Phase Breaker/RConn1 -- Parallel RLC Branch6/LConn1
  Three-Phase Breaker/RConn2 -- Parallel RLC Branch7/LConn1
  Three-Phase Breaker/RConn3 -- Parallel RLC Branch10/LConn1

== system myLibrary/PI_line ==
  Series RLC Branch : spsSeriesRLCBranchLib/Series RLC Branch  LConnTagsString=__new0  RConnTagsString=__new0  BranchType=C  Resistance=1  Inductance=1e-3  SetiL0=off  InitialCurrent=0  Capacitance=T.C  Setx0=on  InitialVoltage=ini.Va1  Measurements=None
  Series RLC Branch1 : spsSeriesRLCBranchLib/Series RLC Branch  LConnTagsString=__new0  RConnTagsString=__new0  BranchType=C  Resistance=1  Inductance=1e-3  SetiL0=off  InitialCurrent=0  Capacitance=T.C  Setx0=on  InitialVoltage=ini.Vb1  Measurements=None
  Series RLC Branch2 : spsSeriesRLCBranchLib/Series RLC Branch  LConnTagsString=__new0  RConnTagsString=__new0  BranchType=C  Resistance=1  Inductance=1e-3  SetiL0=off  InitialCurrent=0  Capacitance=T.C  Setx0=on  InitialVoltage=ini.Vc1  Measurements=None
  Series RLC Branch3 : spsSeriesRLCBranchLib/Series RLC Branch  LConnTagsString=__new0  RConnTagsString=__new0  BranchType=C  Resistance=1  Inductance=1e-3  SetiL0=off  InitialCurrent=0  Capacitance=T.C  Setx0=on  InitialVoltage=ini.Va2  Measurements=None
  Series RLC Branch4 : spsSeriesRLCBranchLib/Series RLC Branch  LConnTagsString=__new0  RConnTagsString=__new0  BranchType=C  Resistance=1  Inductance=1e-3  SetiL0=off  InitialCurrent=0  Capacitance=T.C  Setx0=on  InitialVoltage=ini.Vb2  Measurements=None
  Series RLC Branch5 : spsSeriesRLCBranchLib/Series RLC Branch  LConnTagsString=__new0  RConnTagsString=__new0  BranchType=C  Resistance=1  Inductance=1e-3  SetiL0=off  InitialCurrent=0  Capacitance=T.C  Setx0=on  InitialVoltage=ini.Vc2  Measurements=None
  Series RLC Branch6 : spsSeriesRLCBranchLib/Series RLC Branch  LConnTagsString=__new0  RConnTagsString=__new0  BranchType=RL  Resistance=T.R  Inductance=T.L  SetiL0=off  InitialCurrent=ini.Ia  Capacitance=P.C  Setx0=on  InitialVoltage=P.C  Measurements=None
  Series RLC Branch7 : spsSeriesRLCBranchLib/Series RLC Branch  LConnTagsString=__new0  RConnTagsString=__new0  BranchType=RL  Resistance=T.R  Inductance=T.L  SetiL0=on  InitialCurrent=ini.Ic  Capacitance=P.C  Setx0=on  InitialVoltage=P.C  Measurements=None
  Series RLC Branch8 : spsSeriesRLCBranchLib/Series RLC Branch  LConnTagsString=__new0  RConnTagsString=__new0  BranchType=RL  Resistance=T.R  Inductance=T.L  SetiL0=on  InitialCurrent=ini.Ib  Capacitance=P.C  Setx0=on  InitialVoltage=P.C  Measurements=None
  A1 : PMIOPort  Side=Left
  B1 : PMIOPort  Port=2  Side=Left
  C1 : PMIOPort  Port=3  Side=Left
  A2 : PMIOPort  Port=4  Side=Right
  B2 : PMIOPort  Port=5  Side=Right
  C2 : PMIOPort  Port=6  Side=Right
  connections:
  C2/RConn1 -- Series RLC Branch7/RConn1 -- Series RLC Branch5/LConn1
  B2/RConn1 -- Series RLC Branch8/RConn1 -- Series RLC Branch4/LConn1
  Series RLC Branch3/LConn1 -- Series RLC Branch6/RConn1 -- A2/RConn1
  C1/RConn1 -- Series RLC Branch7/LConn1 -- Series RLC Branch2/LConn1
  Series RLC Branch6/LConn1 -- A1/RConn1 -- Series RLC Branch/LConn1
  Series RLC Branch8/LConn1 -- B1/RConn1 -- Series RLC Branch1/LConn1
  Series RLC Branch2/RConn1 -- Series RLC Branch/RConn1 -- Series RLC Branch1/RConn1
  Series RLC Branch5/RConn1 -- Series RLC Branch4/RConn1 -- Series RLC Branch3/RConn1

== system myLibrary/RL_line ==
  Series RLC Branch6 : spsSeriesRLCBranchLib/Series RLC Branch  LConnTagsString=__new0  RConnTagsString=__new0  BranchType=RL  Resistance=T.R  Inductance=T.L  SetiL0=on  InitialCurrent=ini.Ia  Capacitance=P.C  Setx0=on  InitialVoltage=P.C  Measurements=None
  Series RLC Branch7 : spsSeriesRLCBranchLib/Series RLC Branch  LConnTagsString=__new0  RConnTagsString=__new0  BranchType=RL  Resistance=T.R  Inductance=T.L  SetiL0=on  InitialCurrent=ini.Ic  Capacitance=P.C  Setx0=on  InitialVoltage=P.C  Measurements=None
  Series RLC Branch8 : spsSeriesRLCBranchLib/Series RLC Branch  LConnTagsString=__new0  RConnTagsString=__new0  BranchType=RL  Resistance=T.R  Inductance=T.L  SetiL0=on  InitialCurrent=ini.Ib  Capacitance=P.C  Setx0=on  InitialVoltage=P.C  Measurements=None
  A1 : PMIOPort  Side=Left
  B1 : PMIOPort  Port=2  Side=Left
  C1 : PMIOPort  Port=3  Side=Left
  A2 : PMIOPort  Port=4  Side=Right
  B2 : PMIOPort  Port=5  Side=Right
  C2 : PMIOPort  Port=6  Side=Right
  connections:
  C2/RConn1 -- Series RLC Branch7/RConn1
  Series RLC Branch7/LConn1 -- C1/RConn1
  B1/RConn1 -- Series RLC Branch8/LConn1
  B2/RConn1 -- Series RLC Branch8/RConn1
  A2/RConn1 -- Series RLC Branch6/RConn1
  A1/RConn1 -- Series RLC Branch6/LConn1
